simulink model "Simulations"  (R2021a)
settings: Solver=VariableStepAuto  StartTime=0.0  StopTime=15  RelTol=1e-3
undefined symbols (not defined in the file): Discount_Percentage, GPS_Estimate_Final, GPS_Estimate_Final1, GPS_Estimate_Final2, Item_Prices, Item_Prices1, Item_Prices2, Purchase_Price, PurchasePrices, PurchasePrices1, Shipping, Shipping1, Shipping2
settings Model: Creator=Student  LastModifiedBy=Student

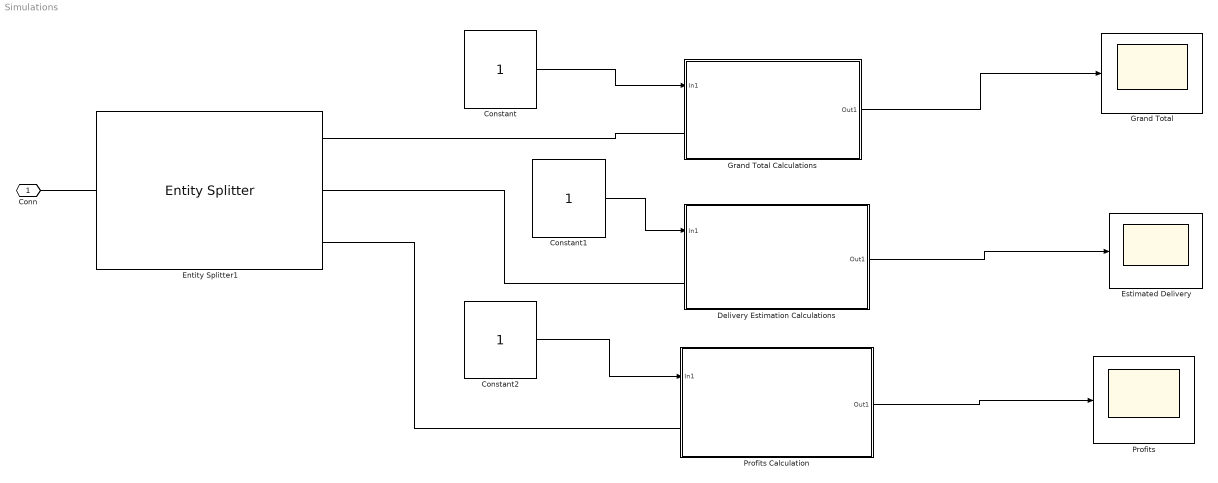
== system Simulations ==
  Constant : Constant
  Constant1 : Constant
  Constant2 : Constant
  Delivery Estimation Calculations : Subsystem
  Entity Splitter1 : EntitySplitter
  Estimated Delivery : Scope
  Grand Total : Scope
  Grand Total Calculations : Subsystem
  Profits : Scope
  Profits Calculation : Subsystem
  Conn : PMIOPort  Side=Left
  wires:
  Grand Total Calculations/1(Out1) -> Grand Total/1
  Constant/1 -> Grand Total Calculations/1(In1)
  Delivery Estimation Calculations/1(Out1) -> Estimated Delivery/1
  Constant1/1 -> Delivery Estimation Calculations/1(In1)
  Profits Calculation/1(Out1) -> Profits/1
  Constant2/1 -> Profits Calculation/1(In1)
  connections:
  Entity Splitter1/RConn1 -- Grand Total Calculations/LConn1
  Entity Splitter1/RConn2 -- Delivery Estimation Calculations/LConn1
  Entity Splitter1/RConn3 -- Profits Calculation/LConn1
  Conn/RConn1 -- Entity Splitter1/LConn1

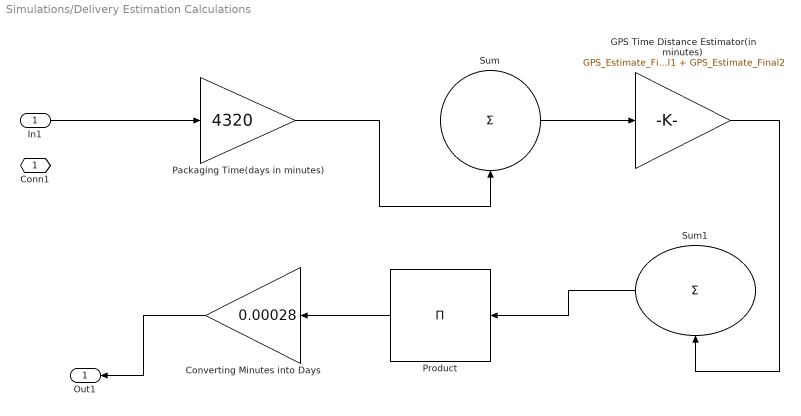
== system Simulations/Delivery Estimation Calculations ==
  In1 : Inport
  Converting Minutes into Days : Gain  Gain=0.00028
  GPS Time Distance Estimator(in minutes) : Gain  Gain=GPS_Estimate_Final + GPS_Estimate_Final1 + GPS_Estimate_Final2
  Packaging Time(days in minutes) : Gain  Gain=4320
  Product : Product  Inputs=1
  Sum : Sum  Inputs=|+
  Sum1 : Sum  Inputs=|+
  Conn1 : PMIOPort  Side=Left
  Out1 : Outport
  wires:
  Converting Minutes into Days/1 -> Out1/1
  Sum/1 -> GPS Time Distance Estimator(in minutes)/1
  GPS Time Distance Estimator(in minutes)/1 -> Sum1/1
  Product/1 -> Converting Minutes into Days/1
  Packaging Time(days in minutes)/1 -> Sum/1
  In1/1 -> Packaging Time(days in minutes)/1
  Sum1/1 -> Product/1

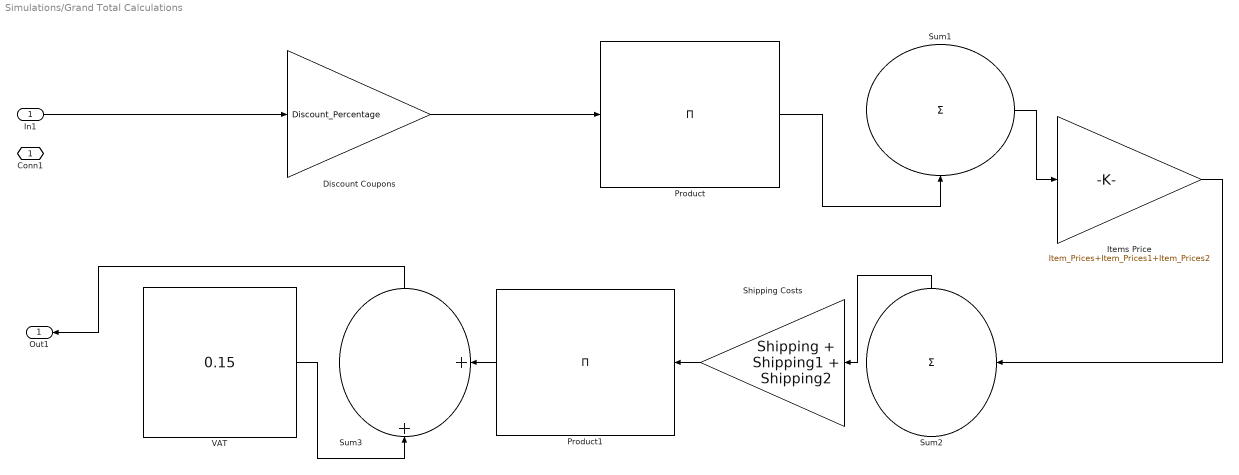
== system Simulations/Grand Total Calculations ==
  In1 : Inport
  Discount Coupons : Gain  Gain=Discount_Percentage
  Items Price : Gain  Gain=Item_Prices+Item_Prices1+Item_Prices2
  Product : Product  Inputs=1
  Product1 : Product  Inputs=1
  Shipping Costs : Gain  Gain=Shipping + Shipping1 + Shipping2
  Sum1 : Sum  Inputs=|+
  Sum2 : Sum  Inputs=|+
  Sum3 : Sum  Inputs=|++
  VAT : Constant  Value=0.15
  Conn1 : PMIOPort  Side=Left
  Out1 : Outport
  wires:
  Shipping Costs/1 -> Product1/1
  Sum1/1 -> Items Price/1
  Product1/1 -> Sum3/2
  Sum2/1 -> Shipping Costs/1
  Items Price/1 -> Sum2/1
  Product/1 -> Sum1/1
  Discount Coupons/1 -> Product/1
  VAT/1 -> Sum3/1
  Sum3/1 -> Out1/1
  In1/1 -> Discount Coupons/1

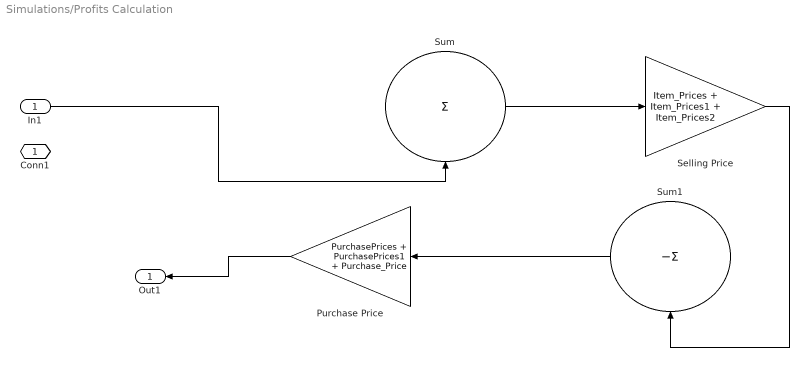
== system Simulations/Profits Calculation ==
  In1 : Inport
  Purchase Price : Gain  Gain=PurchasePrices + PurchasePrices1 + Purchase_Price
  Selling Price : Gain  Gain=Item_Prices + Item_Prices1 + Item_Prices2
  Sum : Sum  Inputs=|+
  Sum1 : Sum  Inputs=|-
  Conn1 : PMIOPort  Side=Left
  Out1 : Outport
  wires:
  Sum/1 -> Selling Price/1
  Purchase Price/1 -> Out1/1
  Sum1/1 -> Purchase Price/1
  Selling Price/1 -> Sum1/1
  In1/1 -> Sum/1
